simulink model "bldc_with_svpwm"  (R2022a)
settings: Solver=FixedStepDiscrete  StartTime=0.0  StopTime=1  RelTol=1e-3
undefined symbols (not defined in the file): Ts, Vdc
libraries: simulink x5, slpidlib x3, spsDCVoltageSourceLib x1, spsPermanentMagnetSynchronousMachineLib x1, spsUniversalBridgeLib x1, spspowerguiLib x1
(part 2 of 2)

== system bldc_with_svpwm/BLDC/SVPWMchen/扇区发波2/Subsystem8/Subsystem ==
  Tx : Inport
  Ty : Inport  Port=2
  Constant1 : Constant  Value=T
  Divide : Product  Inputs=*/
  Divide1 : Product  Inputs=*/
  Gain : Gain  Gain=T
  Gain1 : Gain  Gain=T
  Relational Operator : RelationalOperator  Operator=<=  OutDataTypeStr=boolean  RndMeth=Simplest  InputSameDT=off
  Sum : Sum
  Switch : Switch  Criteria=u2 > Threshold  SaturateOnIntegerOverflow=off  InputSameDT=off
  Switch1 : Switch  Criteria=u2 > Threshold  SaturateOnIntegerOverflow=off  InputSameDT=off
  "Tx " : Outport  VectorParamsAs1DForOutWhenUnconnected=off
  "Ty " : Outport  Port=2  VectorParamsAs1DForOutWhenUnconnected=off
  wires:
  Switch/1 -> "Tx "/1
  Sum/1 -> Relational Operator/1, Divide1/2, Divide/2  "Tx+Ty"
  Tx/1 -> Sum/1, Switch/1, Divide/1  "Tx"
  Relational Operator/1 -> Switch/2, Switch1/2
  Ty/1 -> Sum/2, Divide1/1, Switch1/1
  Divide1/1 -> Gain1/1
  Divide/1 -> Gain/1
  Switch1/1 -> "Ty "/1
  Constant1/1 -> Relational Operator/2
  Gain/1 -> Switch/3
  Gain1/1 -> Switch1/3

== system bldc_with_svpwm/BLDC/SVPWMchen/扇区计算/N=A+2B+4C/A ==
  Vα : Inport
  Vβ : Inport  Port=2
  Gain : Gain  Gain=sqrt(3)
  MATLAB Function : MATLAB Function  TreatAsAtomicUnit=on
  Sign : Signum
  Sum : Sum  Inputs=|+-
  Out1 : Outport
  wires:
  Vα/1 -> Gain/1
  Gain/1 -> Sum/2
  Vβ/1 -> Sum/1
  Sum/1 -> Sign/1
  Sign/1 -> MATLAB Function/1(u)
  MATLAB Function/1(y) -> Out1/1

== system bldc_with_svpwm/BLDC/SVPWMchen/扇区计算/N=A+2B+4C/B ==
  Vα : Inport
  Vβ : Inport  Port=2
  Gain : Gain  Gain=sqrt(3)
  MATLAB Function : MATLAB Function  TreatAsAtomicUnit=on
  Sign : Signum
  Sum : Sum  Inputs=|++
  Out1 : Outport
  wires:
  Sign/1 -> MATLAB Function/1(u)
  Vα/1 -> Gain/1
  Vβ/1 -> Sum/1
  MATLAB Function/1(y) -> Out1/1
  Sum/1 -> Sign/1
  Gain/1 -> Sum/2

== system bldc_with_svpwm/BLDC/SVPWMchen/扇区计算/N=A+2B+4C/C ==
  Vβ : Inport
  MATLAB Function : MATLAB Function  TreatAsAtomicUnit=on
  Sign : Signum
  Out1 : Outport
  wires:
  MATLAB Function/1(y) -> Out1/1
  Sign/1 -> MATLAB Function/1(u)
  Vβ/1 -> Sign/1

== matlab function bldc_with_svpwm/BLDC/Anti_Park/MATLAB Function1 ==
  data: d input; alpha output; q input; angle input
function alpha = fcn(d,q,angle)

alpha = d*cos(angle)-q*sin(angle);

== matlab function bldc_with_svpwm/BLDC/Anti_Park/MATLAB Function2 ==
  data: d input; beta output; q input; angle input
function beta = fcn(d,q,angle)

beta = d*sin(angle)+q*cos(angle);

== matlab function bldc_with_svpwm/BLDC/SVPWMchen/扇区发波2/Subsystem5/MATLAB Function ==
  data: u input; y output
function y = fcn(u)

y = (u(1)-u(2)-u(3))/4;

== matlab function bldc_with_svpwm/BLDC/SVPWMchen/扇区发波2/Subsystem5/MATLAB Function1 ==
  data: u input; y output
function y = fcn(u)

y = (u(1)+u(2)-u(3))/4;

== matlab function bldc_with_svpwm/BLDC/SVPWMchen/扇区发波2/Subsystem5/MATLAB Function2 ==
  data: u input; y output
function y = fcn(u)

y = (u(1)+u(2)+u(3))/4;

== matlab function bldc_with_svpwm/BLDC/SVPWMchen/扇区发波2/Subsystem6/MATLAB Function ==
  data: u input; y output
function y = fcn(u)

y = (u(1)-u(2)-u(3))/4;

== matlab function bldc_with_svpwm/BLDC/SVPWMchen/扇区发波2/Subsystem6/MATLAB Function1 ==
  data: u input; y output
function y = fcn(u)

y = (u(1)+u(2)-u(3))/4;

== matlab function bldc_with_svpwm/BLDC/SVPWMchen/扇区计算/N=A+2B+4C/A/MATLAB Function ==
  data: u input; y output
function y = fcn(u)

y = -0.5*u+0.5;

== matlab function bldc_with_svpwm/BLDC/SVPWMchen/扇区发波2/Subsystem6/MATLAB Function2 ==
  data: u input; y output
function y = fcn(u)

y = (u(1)+u(2)+u(3))/4;

== matlab function bldc_with_svpwm/BLDC/SVPWMchen/扇区发波2/Subsystem7/MATLAB Function ==
  data: u input; y output
function y = fcn(u)

y = (u(1)-u(2)-u(3))/4;

== matlab function bldc_with_svpwm/BLDC/SVPWMchen/扇区发波2/Subsystem7/MATLAB Function1 ==
  data: u input; y output
function y = fcn(u)

y = (u(1)+u(2)-u(3))/4;

== matlab function bldc_with_svpwm/BLDC/SVPWMchen/扇区发波2/Subsystem7/MATLAB Function2 ==
  data: u input; y output
function y = fcn(u)

y = (u(1)+u(2)+u(3))/4;

== matlab function bldc_with_svpwm/BLDC/SVPWMchen/扇区发波2/Subsystem8/MATLAB Function ==
  data: u input; y output
function y = fcn(u)

y = (u(1)-u(2)-u(3))/4;

== matlab function bldc_with_svpwm/BLDC/SVPWMchen/扇区发波2/Subsystem8/MATLAB Function1 ==
  data: u input; y output
function y = fcn(u)

y = (u(1)+u(2)-u(3))/4;

== matlab function bldc_with_svpwm/BLDC/SVPWMchen/扇区发波2/Subsystem8/MATLAB Function2 ==
  data: u input; y output
function y = fcn(u)

y = (u(1)+u(2)+u(3))/4;

== matlab function bldc_with_svpwm/BLDC/SVPWMchen/扇区计算/N=A+2B+4C/C/MATLAB Function ==
  data: u input; y output
function y = fcn(u)

y = 0.5*u+0.5;

== matlab function bldc_with_svpwm/BLDC/SVPWMchen/扇区发波2/Subsystem4/MATLAB Function ==
  data: u input; y output
function y = fcn(u)

y = (u(1)-u(2)-u(3))/4;

== matlab function bldc_with_svpwm/BLDC/SVPWMchen/扇区发波2/Subsystem4/MATLAB Function1 ==
  data: u input; y output
function y = fcn(u)

y = (u(1)+u(2)-u(3))/4;

== matlab function bldc_with_svpwm/BLDC/SVPWMchen/扇区发波2/Subsystem4/MATLAB Function2 ==
  data: u input; y output
function y = fcn(u)

y = (u(1)+u(2)+u(3))/4;

== matlab function bldc_with_svpwm/BLDC/Park_Trans/MATLAB Function ==
  data: alpha input; q output; beta input; angle input
function q = fcn(alpha,beta,angle)

q = -alpha*sin(angle)+beta*cos(angle);

== matlab function bldc_with_svpwm/BLDC/Park_Trans/MATLAB Function1 ==
  data: alpha input; d output; beta input; angle input
function d = fcn(alpha,beta,angle)

d = alpha*cos(angle)+beta*sin(angle);

== matlab function bldc_with_svpwm/BLDC/Clark_Trans/MATLAB Function ==
  data: u input; alpha output; v input; w input
function alpha = fcn(u,v,w)

alpha = (2/3)*(u+(-1/2)*v+(-1/2)*w);

== matlab function bldc_with_svpwm/BLDC/SVPWMchen/扇区发波2/Subsystem2/MATLAB Function ==
  data: u input; y output
function y = fcn(u)

y = (u(1)-u(2)-u(3))/4;

== matlab function bldc_with_svpwm/BLDC/SVPWMchen/扇区发波2/Subsystem2/MATLAB Function1 ==
  data: u input; y output
function y = fcn(u)

y = (u(1)+u(2)-u(3))/4;

== matlab function bldc_with_svpwm/BLDC/SVPWMchen/扇区计算/N=A+2B+4C/B/MATLAB Function ==
  data: u input; y output
function y = fcn(u)

y = -0.5*u+0.5;

== matlab function bldc_with_svpwm/BLDC/SVPWMchen/扇区发波2/Subsystem2/MATLAB Function2 ==
  data: u input; y output
function y = fcn(u)

y = (u(1)+u(2)+u(3))/4;

== matlab function bldc_with_svpwm/BLDC/Clark_Trans/MATLAB Function1 ==
  data: beta output; v input; w input
function beta = fcn(v,w)

beta = (2/3)*((sqrt(3)/2)*v+(-sqrt(3)/2)*w);
